simulink model "module1example"  (R2022b)
settings: Solver=FixedStepAuto  StartTime=0.0  StopTime=20  FixedStep=0.1  RelTol=1e-3
model workspace (MAT data in the model file):
  amp = 1
  sysamp = 1
  sysfreq = 1
undefined symbols (not defined in the file): useramp
settings Model: Creator=nnakhjiri  LastModifiedBy=nnakhjiri

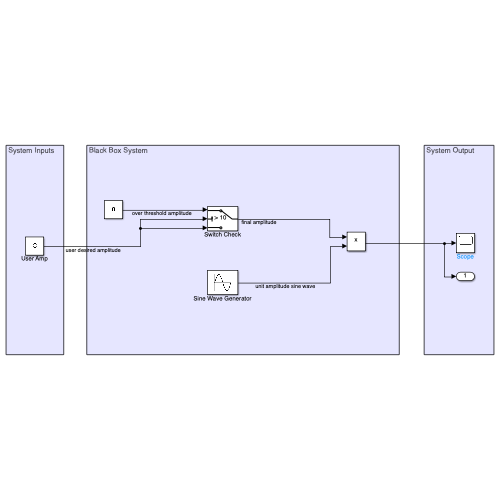
[thumbnail: Simulink's stored preview of the top-level diagram]
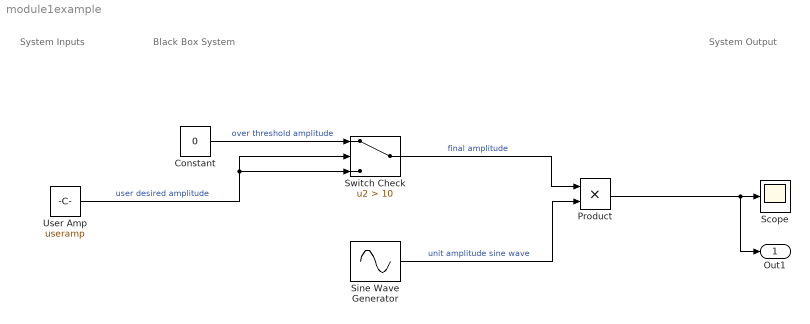
== system module1example ==
  note: System Output
  note: Black Box System
  note: System Inputs
  Constant : Constant  Value=0
  Product : Product
  Scope : Scope
  Sine Wave Generator : Sin  SampleTime=0
  Switch Check : Switch  Criteria=u2 > Threshold  Threshold=10  SaturateOnIntegerOverflow=off  InputSameDT=off
  User Amp : Constant  Value=useramp
  Out1 : Outport
  wires:
  User Amp/1 -> Switch Check/3, Switch Check/2  "user desired amplitude"
  Switch Check/1 -> Product/1  "final amplitude"
  Sine Wave Generator/1 -> Product/2  "unit amplitude sine wave"
  Product/1 -> Out1/1, Scope/1
  Constant/1 -> Switch Check/1  "over threshold amplitude"
